simulink model "plantPWM"  (R2022b)
settings: Solver=ode15s  StartTime=0.0  StopTime=10.0  RelTol=1e-3  EnableMultiTasking=on
PreLoadFcn:
  | % Parameters
  | etc_plant_data;
  | Fs = 1000;
values from neighbouring files (symbols this model uses):
  J = 0.000245    [allParamValues.mat]
libraries: simulink x1
settings Model: Creator=nicholas  LastModifiedBy=bensweet
settings SolverCC: MaxConsecutiveZCs=25  AlgebraicLoopSolver=TrustRegion
settings DataIOCC: LimitDataPoints=on  SaveFormat=Array  ReturnWorkspaceOutputs=off
settings OptimizationCC: DefaultParameterBehavior=Inlined  ExpressionDepthLimit=2147483647  InitFltsAndDblsToZero=on  LifeSpan=inf
settings DebuggingCC: UnconnectedInputMsg=warning  UnconnectedOutputMsg=warning  UnconnectedLineMsg=warning  PregeneratedLibrarySubsystemCodeDiagnostic=none  SFMachineParentedDataDiag=warning
settings HardwareCC: ProdBitPerPointer=32  ProdBitPerSizeT=32  ProdBitPerPtrDiffT=32  ProdLargestAtomicFloat=None  ProdIntDivRoundTo=Undefined  ProdEndianess=Unspecified  ProdWordSize=32  ProdHWDeviceType=32-bit Generic
settings ModelReferenceCC: EnableRefExpFcnMdlSchedulingChecks=on  ModelReferenceMinAlgLoopOccurrences=on  PropagateSignalLabelsOutOfModel=off
settings SFSimCC: SimUseLocalCustomCode=off
settings RTWCC: RTWUseLocalCustomCode=off  DLArmComputeVersion=19.05
settings CodeAppCC: StateflowObjectComments=on
settings GRTTargetCC: TargetLangStandard=C89/C90 (ANSI)  CombineOutputUpdateFcns=off  GRTInterface=on
settings ConfigComp: CovMetricSettings=dw  CovSaveCumulativeToWorkspaceVar=on  CovSaveSingleToWorkspaceVar=on  CovExternalEMLEnable=off  CovSFcnEnable=off

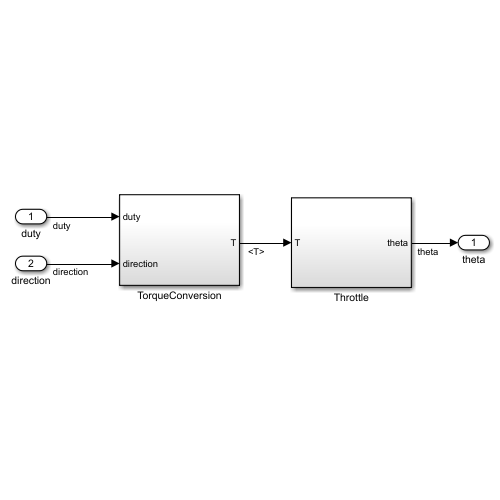
[thumbnail: Simulink's stored preview of the top-level diagram]
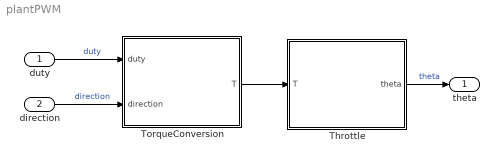
== system plantPWM ==
  duty : Inport
  direction : Inport  Port=2
  Throttle : Subsystem
  TorqueConversion : Subsystem
  theta : Outport  VectorParamsAs1DForOutWhenUnconnected=off
  wires:
  duty/1 -> TorqueConversion/1(duty)  "duty"
  direction/1 -> TorqueConversion/2(direction)  "direction"
  TorqueConversion/1(T) -> Throttle/1(T)
  Throttle/1(theta) -> theta/1  "theta"

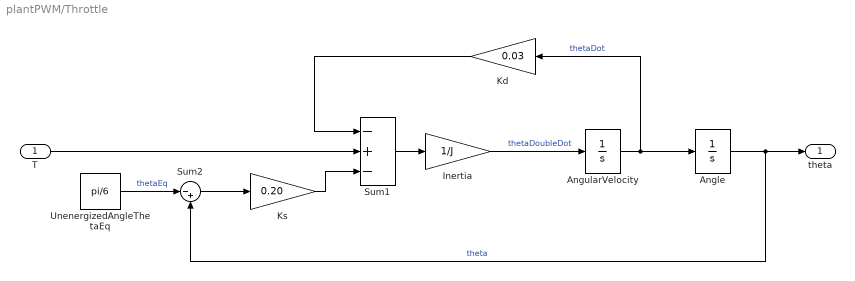
== system plantPWM/Throttle ==
  T : Inport
  Angle : Integrator  InitialCondition=pi/6  LimitOutput=on  UpperSaturationLimit=pi/2  LowerSaturationLimit=0
      settings: AttributesFormatString=Initial condition: %<InitialCondition>\n%<LowerSaturationLimit> <= theta <= %<UpperSaturationLimit>
  AngularVelocity : Integrator
      settings: AttributesFormatString=Initial condition: %<InitialCondition>
  Inertia : Gain  Gain=1/J  SaturateOnIntegerOverflow=on  OutDataTypeStr=Inherit: Same as input  ParamDataTypeStr=Inherit: Same as input
  Kd : Gain  Gain=0.03  SaturateOnIntegerOverflow=on  OutDataTypeStr=Inherit: Same as input  ParamDataTypeStr=Inherit: Same as input
  Ks : Gain  Gain=0.20  SaturateOnIntegerOverflow=on  OutDataTypeStr=Inherit: Same as input  ParamDataTypeStr=Inherit: Same as input
  Sum1 : Sum  Inputs=-+-  SaturateOnIntegerOverflow=on
  Sum2 : Sum  Inputs=|-+  SaturateOnIntegerOverflow=on
  UnenergizedAngleThetaEq : Constant  Value=pi/6
  theta : Outport  VectorParamsAs1DForOutWhenUnconnected=off
  wires:
  Sum1/1 -> Inertia/1
  Inertia/1 -> AngularVelocity/1  "thetaDoubleDot"
  Kd/1 -> Sum1/1
  Sum2/1 -> Ks/1
  Ks/1 -> Sum1/3
  UnenergizedAngleThetaEq/1 -> Sum2/1  "thetaEq"
  Angle/1 -> theta/1, Sum2/2  "theta"
  AngularVelocity/1 -> Angle/1, Kd/1  "thetaDot"
  T/1 -> Sum1/2

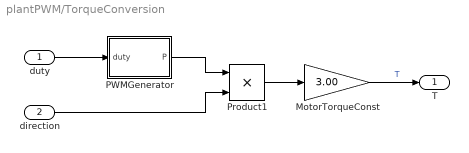
== system plantPWM/TorqueConversion ==
  duty : Inport
  direction : Inport  Port=2
  MotorTorqueConst : Gain  Gain=3.00  SaturateOnIntegerOverflow=on  OutDataTypeStr=Inherit: Same as input  ParamDataTypeStr=Inherit: Same as input
  PWMGenerator : Subsystem  DialogController=POWERSYS.PowerSysDialog
  Product1 : Product  SaturateOnIntegerOverflow=on  OutDataTypeStr=Inherit: Same as first input
  T : Outport  VectorParamsAs1DForOutWhenUnconnected=off
  wires:
  duty/1 -> PWMGenerator/1(duty)
  MotorTorqueConst/1 -> T/1  "T"
  direction/1 -> Product1/2
  Product1/1 -> MotorTorqueConst/1
  PWMGenerator/1(P) -> Product1/1

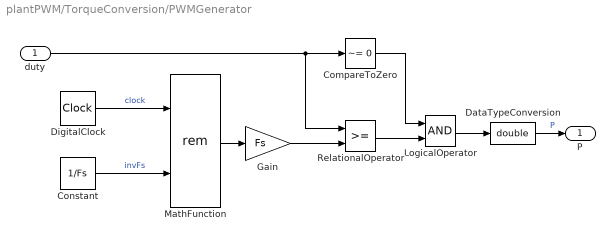
== system plantPWM/TorqueConversion/PWMGenerator ==
  duty : Inport
  CompareToZero : simulink/Logic and Bit Operations/Compare To Zero  relop=~=  OutDataTypeStr=boolean
  Constant : Constant  Value=1/Fs  SampleTime=0
  DataTypeConversion : DataTypeConversion  OutDataTypeStr=double  SaturateOnIntegerOverflow=off  RndMeth=Floor
  DigitalClock : DigitalClock  SampleTime=1/(50*Fs)
      settings: AttributesFormatString=Ts = %<SampleTime>
  Gain : Gain  Gain=Fs  SaturateOnIntegerOverflow=on  OutDataTypeStr=Inherit: Same as input  ParamDataTypeStr=Inherit: Same as input
  LogicalOperator : Logic  AllPortsSameDT=off  OutDataTypeStr=boolean
  MathFunction : Math  Operator=rem  SignedPower=on
  RelationalOperator : RelationalOperator  OutDataTypeStr=boolean  InputSameDT=off
  P : Outport  VectorParamsAs1DForOutWhenUnconnected=off
  wires:
  duty/1 -> CompareToZero/1, RelationalOperator/1
  RelationalOperator/1 -> LogicalOperator/2
  CompareToZero/1 -> LogicalOperator/1
  LogicalOperator/1 -> DataTypeConversion/1
  DataTypeConversion/1 -> P/1  "P"
  Gain/1 -> RelationalOperator/2
  MathFunction/1 -> Gain/1
  Constant/1 -> MathFunction/2  "invFs"
  DigitalClock/1 -> MathFunction/1  "clock"
